simulink model "LQR_lp2"  (R2021a)
settings: Solver=ode4  StartTime=0.0  StopTime=inf  FixedStep=0.001  RelTol=1e-3
libraries: ETlabLibrary x5, simulink x2
settings Model: SimulationMode=external  Creator=Administrator  LastModifiedBy=ETLAB
settings SolverCC: AlgebraicLoopSolver=TrustRegion  DecoupledContinuousIntegration=on  MinimalZcImpactIntegration=on
settings DataIOCC: ReturnWorkspaceOutputs=off
settings DebuggingCC: SFMachineParentedDataDiag=warning  ArithmeticOperatorsInVariantConditions=warning
settings SFSimCC: SimUseLocalCustomCode=off  CustomCodeUndefinedFunction=UseInterfaceOnly
settings RTWCC: Description=Simulink Desktop Real-Time  SystemTargetFile=sldrt.tlc  TemplateMakefile=sldrt.tmf  RTWUseLocalCustomCode=off  RTWCompilerOptimization=on
settings CodeAppCC: MaxIdLength=95
settings SimulinkDesktopRealTimeCC: TargetPreCompLibLocation=D:\MATLAB2021a\toolbox\sldrt\lib\win64

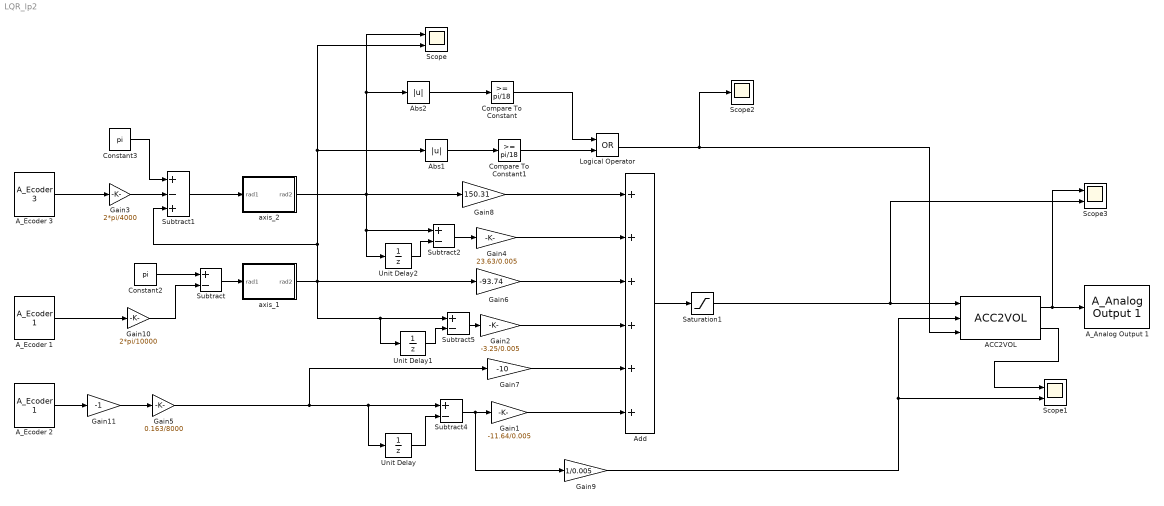
== system LQR_lp2 ==
  ACC2VOL : ETlabLibrary/ACC2VOL  PGain=0.18  IGain=27  VelocityUpper=0.6  VelocityLower=-0.6  VoltageUpper=2  VoltageLower=-2  Ts=0.005
      settings: SourceProductName=ETlabLibrary
  A_Analog Output 1 : ETlabLibrary/A_Analog Output 1  SampleTime=0.005
      settings: SourceProductName=ETlabLibrary
  A_Ecoder 1 : ETlabLibrary/A_Ecoder 1  SampleTime=0.005
      settings: SourceProductName=ETlabLibrary
  A_Ecoder 2 : ETlabLibrary/A_Ecoder 1  SampleTime=0.005
      link override Encoder 01: SampleTime=SampleTime  MaxMissedTicks=10000000  ShowMissedTicks=off  YieldWhenWaiting=on  DrvName=National_Instruments/PCI-6229  DrvAddress=4294967295  DrvOptions=[0 0 0 2 2]  Channels=1  QuadMode=3  IndexPulse=1  InputFilter=Inf  DataType=1
      link override Encoder Input4: SampleTime=SampleTime  MaxMissedTicks=1000000  ShowMissedTicks=off  YieldWhenWaiting=off  DrvName=National_Instruments/PCI-6602  DrvAddress=4294967295  DrvOptions=[255 3 3 3 2 2 2 2 2]  Channels=5  QuadMode=3  IndexPulse=2  InputFilter=Inf  DataType=1
      settings: SourceProductName=ETlabLibrary
  A_Ecoder 3 : ETlabLibrary/A_Ecoder 3  SampleTime=0.01
      settings: SourceProductName=ETlabLibrary
  Abs1 : Abs
  Abs2 : Abs
  Add : Sum  Inputs=++++++
  Compare To Constant : simulink/Logic and Bit Operations/Compare To Constant  relop=>=  const=pi/18  OutDataTypeStr=boolean
  Compare To Constant1 : simulink/Logic and Bit Operations/Compare To Constant  relop=>=  const=pi/18  OutDataTypeStr=boolean
  Constant2 : Constant  Value=pi
  Constant3 : Constant  Value=pi
  Gain1 : Gain  Gain=-11.64/0.005  OutDataTypeStr=double
  Gain10 : Gain  Gain=2*pi/10000  OutDataTypeStr=double
  Gain11 : Gain  Gain=-1  OutDataTypeStr=double
  Gain2 : Gain  Gain=-3.25/0.005  OutDataTypeStr=double
  Gain3 : Gain  Gain=2*pi/4000  OutDataTypeStr=double
  Gain4 : Gain  Gain=23.63/0.005  OutDataTypeStr=double
  Gain5 : Gain  Gain=0.163/8000  OutDataTypeStr=double
  Gain6 : Gain  Gain=-93.74  OutDataTypeStr=double
  Gain7 : Gain  Gain=-10  OutDataTypeStr=double
  Gain8 : Gain  Gain=150.31  OutDataTypeStr=double
  Gain9 : Gain  Gain=1/0.005  OutDataTypeStr=double
  Logical Operator : Logic  Operator=OR  AllPortsSameDT=off  OutDataTypeStr=boolean
  Saturation1 : Saturate  UpperLimit=30  LowerLimit=-30
  Scope : Scope  NumInputPorts=2
  Scope1 : Scope  NumInputPorts=2
  Scope2 : Scope
  Scope3 : Scope  NumInputPorts=2
  Subtract{,2,4..5} (4 alike) : Sum  Inputs=+-
  Subtract1 : Sum  Inputs=+-+
  Unit Delay : UnitDelay  SampleTime=0.005  HasFrameUpgradeWarning=on
  Unit Delay1 : UnitDelay  SampleTime=0.005  HasFrameUpgradeWarning=on
  Unit Delay2 : UnitDelay  SampleTime=0.005  HasFrameUpgradeWarning=on
  axis_1 : MATLAB Function  TreatAsAtomicUnit=on
  axis_2 : MATLAB Function  TreatAsAtomicUnit=on
  wires:
  Constant2/1 -> Subtract/1
  Subtract/1 -> axis_1/1(rad1)
  Gain10/1 -> Subtract/2
  Subtract4/1 -> Gain9/1, Gain1/1
  Gain5/1 -> Unit Delay/1, Subtract4/1, Gain7/1
  Unit Delay/1 -> Subtract4/2
  Subtract5/1 -> Gain2/1
  axis_1/1(rad2) -> Scope/2, Abs1/1, Subtract1/3, Subtract5/1, Unit Delay1/1, Gain6/1
  Unit Delay1/1 -> Subtract5/2
  A_Ecoder 2/1 -> Gain11/1
  A_Ecoder 1/1 -> Gain10/1
  Gain11/1 -> Gain5/1
  Add/1 -> Saturation1/1
  Saturation1/1 -> Scope3/2, ACC2VOL/1
  Gain9/1 -> Scope1/2, ACC2VOL/2
  ACC2VOL/1 -> Scope3/1, A_Analog Output 1/1
  Subtract1/1 -> axis_2/1(rad1)
  Constant3/1 -> Subtract1/1
  A_Ecoder 3/1 -> Gain3/1
  Gain3/1 -> Subtract1/2
  Subtract2/1 -> Gain4/1
  axis_2/1(rad2) -> Scope/1, Abs2/1, Gain8/1, Subtract2/1, Unit Delay2/1
  Unit Delay2/1 -> Subtract2/2
  Abs2/1 -> Compare To Constant/1
  Abs1/1 -> Compare To Constant1/1
  Compare To Constant/1 -> Logical Operator/1
  Compare To Constant1/1 -> Logical Operator/2
  Gain1/1 -> Add/6
  Gain7/1 -> Add/5
  Gain2/1 -> Add/4
  Gain6/1 -> Add/3
  Gain4/1 -> Add/2
  Gain8/1 -> Add/1
  Logical Operator/1 -> Scope2/1, ACC2VOL/3
  ACC2VOL/2 -> Scope1/1

== matlab function LQR_lp2/axis_1 ==
  data: rad1 input; rad2 output
function rad2 = ChangeRad(rad1)

while(rad1>pi)
    rad1 = rad1 - 2 * pi;
end
while(rad1<-pi)
    rad1 = rad1 + 2 * pi;
end

rad2 = rad1;

== matlab function LQR_lp2/axis_2 ==
  data: rad1 input; rad2 output
function rad2 = ChangeRad(rad1)

while(rad1>pi)
    rad1 = rad1 - 2 * pi;
end
while(rad1<-pi)
    rad1 = rad1 + 2 * pi;
end

rad2 = rad1;
